simulink model "follow_path"  (R2017a)
settings: Solver=FixedStepAuto  StartTime=0.0  StopTime=200  FixedStep=0.001  RelTol=1e-3
settings Model: Creator=Administrator  LastModifiedBy=Administrator
settings DataIOCC: ExternalInput=[times]

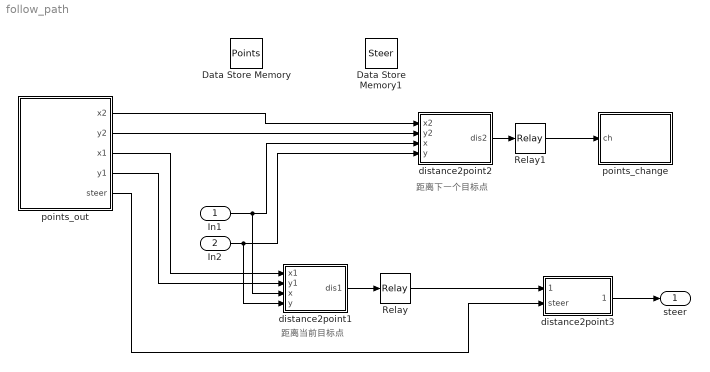
== system follow_path ==
  note: 距离下一个目标点
  note: 距离当前目标点
  In1 : Inport
  In2 : Inport  Port=2
  Data Store Memory : DataStoreMemory  DataStoreName=Points  ReadBeforeWriteMsg=warning  WriteAfterWriteMsg=warning  WriteAfterReadMsg=warning  InitialValue=1  ShowAdditionalParam=off  OutDataTypeStr=double
  Data Store Memory1 : DataStoreMemory  DataStoreName=Steer  ReadBeforeWriteMsg=warning  WriteAfterWriteMsg=warning  WriteAfterReadMsg=warning  ShowAdditionalParam=off  OutDataTypeStr=double
  Relay : Relay  OnSwitchValue=1  OffSwitchValue=0.5
  Relay1 : Relay  OnSwitchValue=1.5  OffSwitchValue=0.2
  distance2point1 : MATLAB Function  TreatAsAtomicUnit=on
  distance2point2 : MATLAB Function  TreatAsAtomicUnit=on
  distance2point3 : MATLAB Function  TreatAsAtomicUnit=on
  points_change : MATLAB Function  TreatAsAtomicUnit=on
  points_out : MATLAB Function  TreatAsAtomicUnit=on
  steer : Outport
  wires:
  distance2point1/1(dis1) -> Relay/1
  Relay/1 -> distance2point3/1(steer_ch)
  distance2point2/1(dis2) -> Relay1/1
  Relay1/1 -> points_change/1(ch)
  points_out/1(x2) -> distance2point2/1(x2)
  points_out/2(y2) -> distance2point2/2(y2)
  In1/1 -> distance2point1/3(x), distance2point2/3(x)
  In2/1 -> distance2point1/4(y), distance2point2/4(y)
  points_out/3(x1) -> distance2point1/1(x1)
  points_out/4(y1) -> distance2point1/2(y1)
  points_out/5(steer) -> distance2point3/2(steer)
  distance2point3/1(steer_out) -> steer/1

== matlab function follow_path/distance2point3 ==
  data: steer_ch input; steer input; Steer data_store_memory; steer_out output
function steer_out = fcn(steer_ch, steer)
global Steer;
if steer_ch > 0
    Steer = steer;
end
steer_out = Steer;

== matlab function follow_path/points_change ==
  data: ch input; Points data_store_memory
function fcn(ch)
global Points;
if ch > 0 && Points < 2
    Points = Points + 1;
end

== matlab function follow_path/distance2point1 ==
  data: x1 input; dis1 output; y1 input; x input; y input
function dis1 = fcn(x1, y1, x, y)
dis1 = sqrt((x1-x)^2 + (y1-y)^2);

== matlab function follow_path/distance2point2 ==
  data: x2 input; dis2 output; y2 input; x input; y input
function dis2 = fcn(x2, y2, x, y)
dis2 = sqrt((x2-x)^2 + (y2-y)^2);

== matlab function follow_path/points_out ==
  data: x2 output; y2 output; x1 output; y1 output; steer output; Points data_store_memory
function [ x2, y2, x1, y1, steer] = fcn
global Points;
i = 0;
i = Points;
points = [1 2 3; 5 6 7; 7 8 9];
x1 = points(i,1);
y1 = points(i,2);
steer = points(i,3);
x2 = points(i+1,1);
y2 = points(i+1,2);
